simulink model "smo_basic"  (R2025a)
settings: Solver=ode1  StartTime=0.0  StopTime=10.0  FixedStep=1e-5  RelTol=1e-3
undefined symbols (not defined in the file): Ke, Kslide, L, omega, R, Vamp
settings Model: Creator=86156  LastModifiedBy=86156

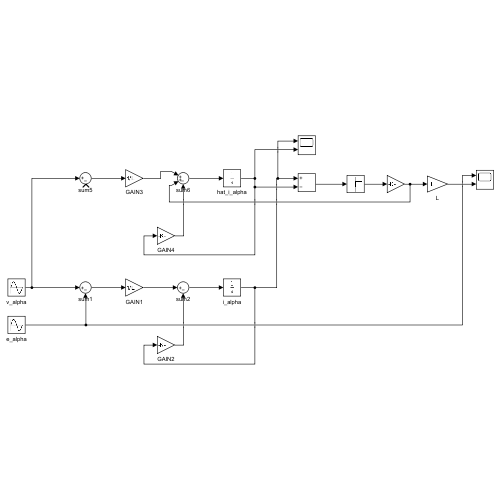
[thumbnail: Simulink's stored preview of the top-level diagram]
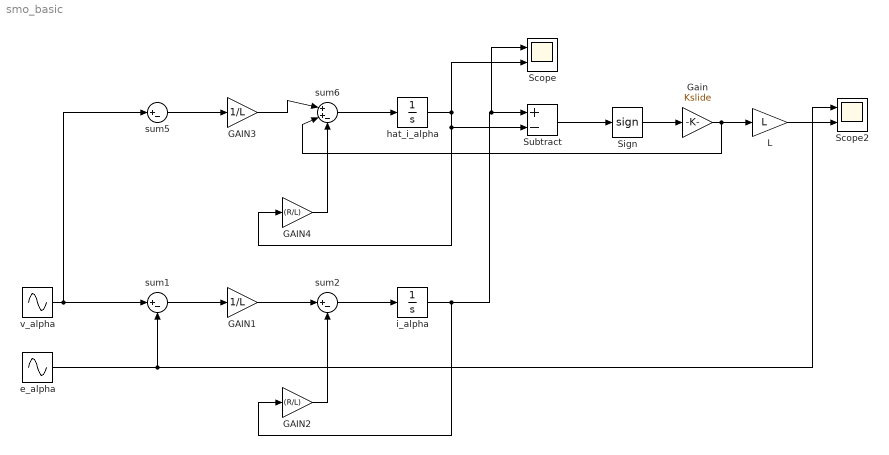
== system smo_basic ==
  GAIN1 : Gain  Gain=1/L
  GAIN2 : Gain  Gain=(R/L)
  GAIN3 : Gain  Gain=1/L
  GAIN4 : Gain  Gain=(R/L)
  Gain : Gain  Gain=Kslide
  L : Gain  Gain=L
  Scope : Scope  NumInputPorts=2
      settings: ActiveDisplayYMinimum=-1  ActiveDisplayYMaximum=1
  Scope2 : Scope  NumInputPorts=2
      settings: ActiveDisplayYMinimum=-23.217659339501441  ActiveDisplayYMaximum=31.907340655566745  DataLoggingVariableName=ScopeData2
  Sign : Signum
  Subtract : Sum  Inputs=+-
  e_alpha : Sin  Amplitude=Ke*omega  Frequency=omega  Phase=pi  SampleTime=0
  hat_i_alpha : Integrator  InitialCondition=0.001
  i_alpha : Integrator
  sum1 : Sum  Inputs=|+-
  sum2 : Sum  Inputs=|+-
  sum5 : Sum  Inputs=|+-
  sum6 : Sum  Inputs=|++-
  v_alpha : Sin  Amplitude=Vamp  Frequency=omega  SampleTime=0
  wires:
  e_alpha/1 -> sum1/2, Scope2/1
  sum1/1 -> GAIN1/1
  GAIN1/1 -> sum2/1
  GAIN2/1 -> sum2/2
  i_alpha/1 -> Scope/1, Subtract/1, GAIN2/1
  sum2/1 -> i_alpha/1
  v_alpha/1 -> sum1/1, sum5/1
  hat_i_alpha/1 -> Subtract/2, GAIN4/1, Scope/2
  sum6/1 -> hat_i_alpha/1
  GAIN3/1 -> sum6/1
  sum5/1 -> GAIN3/1
  Subtract/1 -> Sign/1
  L/1 -> Scope2/2
  GAIN4/1 -> sum6/3
  Sign/1 -> Gain/1
  Gain/1 -> sum6/2, L/1
